simulink model "project_2023_11_6_p50"  (R2021b)
settings: Solver=ode5  StartTime=0.0  StopTime=100.0  FixedStep=0.1  RelTol=1e-3
settings Model: Creator=yingguang wang  LastModifiedBy=yingguang wang
settings HardwareCC: ProdHWDeviceType=AMD->x86-64 (Windows64)
settings SFSimCC: SimTargetLang=C++

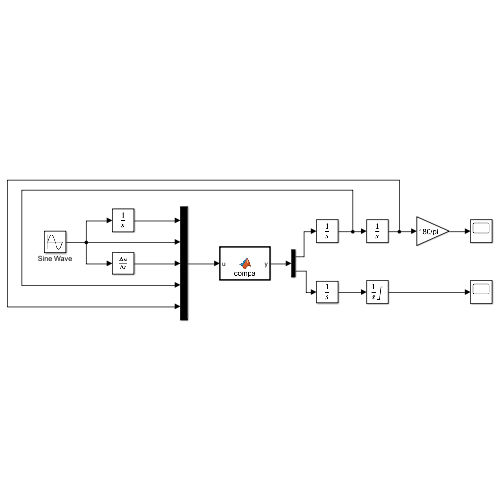
[thumbnail: Simulink's stored preview of the top-level diagram]
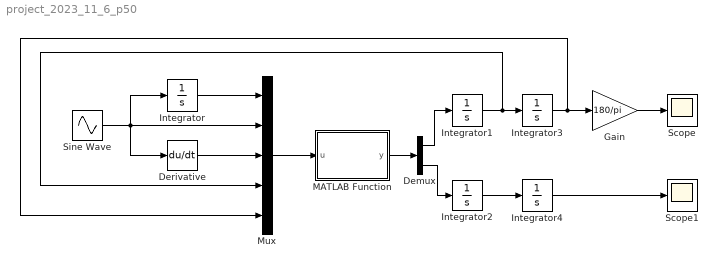
== system project_2023_11_6_p50 ==
  Demux : Demux  Outputs=2
  Derivative : Derivative
  Gain : Gain  Gain=180/pi
  Integrator{,1..3} (4 alike) : Integrator
  Integrator4 : Integrator  InitialCondition=70  LimitOutput=on  UpperSaturationLimit=70  LowerSaturationLimit=40  IgnoreLimit=on
  MATLAB Function : MATLAB Function  TreatAsAtomicUnit=on
  Mux : Mux  Inputs=5
  Scope : Scope
  Scope1 : Scope
  Sine Wave : Sin  Frequency=0.2  SampleTime=0
  wires:
  Sine Wave/1 -> Integrator/1, Derivative/1, Mux/2
  Integrator/1 -> Mux/1
  Derivative/1 -> Mux/3
  Mux/1 -> MATLAB Function/1(u)
  Integrator1/1 -> Mux/4, Integrator3/1
  Integrator2/1 -> Integrator4/1
  Integrator3/1 -> Gain/1, Mux/5
  Gain/1 -> Scope/1
  Integrator4/1 -> Scope1/1
  MATLAB Function/1(y) -> Demux/1
  Demux/1 -> Integrator1/1
  Demux/2 -> Integrator2/1

== matlab function project_2023_11_6_p50/MATLAB Function ==
  data: u input size=5; y output
function y = compa(u)
r1 = 15;
r2 = 55;
a = [r2 * sin(u(5)) 1; 
     r2 * cos(u(5)) 0];
b = [-r1 * u(2)^2 * cos(u(1)) - r2 * u(4)^2*cos(u(5)) - r1 * u(3) * sin(u(1));
    r1 * u(2)^2*sin(u(1))-r1 * u(3) * cos(u(1)) + r2 * u(4)^2 * sin(u(5))];
x = inv(a) * b;
y = x;
